simulink model "F550_Models"  (R2024a)
settings: Solver=ode4  StartTime=0.0  StopTime=10.0  FixedStep=0.01  RelTol=1e-3
settings Model: Creator=UASG  LastModifiedBy=UASG

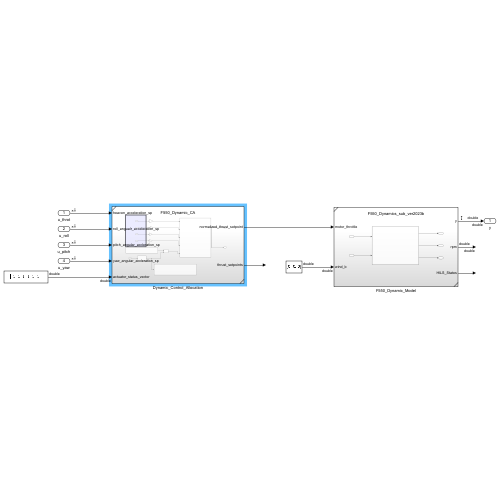
[thumbnail: Simulink's stored preview of the top-level diagram]
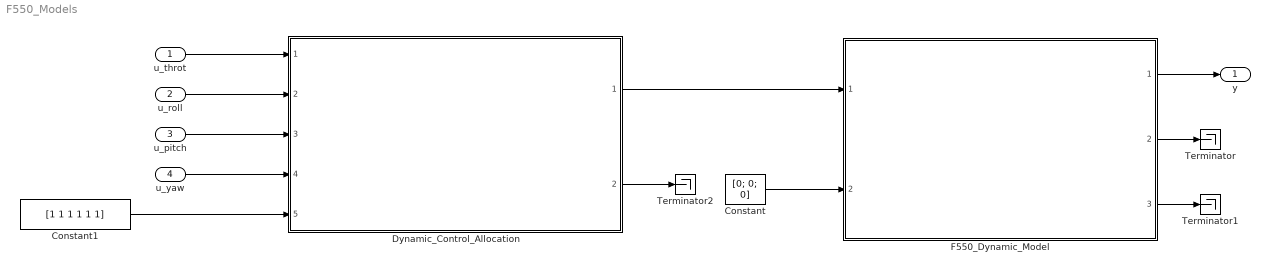
== system F550_Models ==
  u_throt : Inport
  u_roll : Inport  Port=2
  u_pitch : Inport  Port=3
  u_yaw : Inport  Port=4
  Constant : Constant  Value=[0; 0; 0]
  Constant1 : Constant  Value=[1 1 1 1 1 1]
  Dynamic_Control_Allocation : Subsystem  ReferencedSubsystem=F550_Dynamic_CA
  F550_Dynamic_Model : Subsystem  ReferencedSubsystem=F550_Dynamics_sub_ver2023b
  Terminator : Terminator
  Terminator1 : Terminator
  Terminator2 : Terminator
  y : Outport
  wires:
  Constant/1 -> F550_Dynamic_Model/2
  F550_Dynamic_Model/2 -> Terminator/1
  F550_Dynamic_Model/3 -> Terminator1/1
  F550_Dynamic_Model/1 -> y/1
  u_throt/1 -> Dynamic_Control_Allocation/1
  u_pitch/1 -> Dynamic_Control_Allocation/3
  u_roll/1 -> Dynamic_Control_Allocation/2
  u_yaw/1 -> Dynamic_Control_Allocation/4
  Dynamic_Control_Allocation/1 -> F550_Dynamic_Model/1
  Constant1/1 -> Dynamic_Control_Allocation/5
  Dynamic_Control_Allocation/2 -> Terminator2/1
